simulink library "inp"  (R2021b)
settings: Solver=VariableStepAuto  StartTime=0.0  StopTime=10.0  RelTol=1e-3
undefined symbols (not defined in the file): C_TASK_5MS_S, FALSE, KINP_AcoreReadyToSlp_flg_ovrdflg, KINP_AcoreReadyToSlp_flg_ovrdval, KINP_AllowMovThd_OTA_enum_ovrdflg, KINP_AllowMovThd_OTA_enum_ovrdval, KINP_APSAngleTarget_Deg_ovrdflg, KINP_APSAngleTarget_Deg_ovrdval, KINP_APSDecReq_mps2_ovrdflg, KINP_APSDecReq_mps2_ovrdval, KINP_APSDecReqA_flg_ovrdflg, KINP_APSDecReqA_flg_ovrdval, KINP_APSDFLL_cm_ovrdflg, KINP_APSDFLL_cm_ovrdval, KINP_APSDFLR_cm_ovrdflg, KINP_APSDFLR_cm_ovrdval, KINP_APSDRLL_cm_ovrdflg, KINP_APSDRLL_cm_ovrdval, KINP_APSDRLR_cm_ovrdflg, KINP_APSDRLR_cm_ovrdval, KINP_APSExitCondition_enum_ovrdflg, KINP_APSExitCondition_enum_ovrdval, KINP_APSHWVer_enum_ovrdflg, KINP_APSHWVer_enum_ovrdval, KINP_APSProgressPCT_pct_ovrdflg, KINP_APSProgressPCT_pct_ovrdval, KINP_APSReq_enum_ovrdflg, KINP_APSReq_enum_ovrdval, KINP_APSRQDisplay_enum_ovrdflg, KINP_APSRQDisplay_enum_ovrdval, KINP_APSRqEPASCtrl_flg_ovrdflg, KINP_APSRqEPASCtrl_flg_ovrdval, KINP_APSShiftPosnReq_enum_ovrdval, KINP_APSShiftPosnReq_enum_ovrflg, KINP_APSSpeedCMD_kph_ovrdval, KINP_APSSpeedCMD_kph_ovrflg, KINP_APSStaSystem_enum_ovrdflg, KINP_APSStaSystem_enum_ovrdval, KINP_APSSWVer_enum_ovrdflg, KINP_APSSWVer_enum_ovrdval, KINP_APSVMCReqA_flg_ovrdval, KINP_APSVMCReqA_flg_ovrflg, KINP_APSVRqEPASCtrl_flg_ovrdflg, KINP_APSVRqEPASCtrl_flg_ovrdval, KINP_AuxBattVolmV_mV_ovrdflg, KINP_AuxBattVolmV_mV_ovrdval, KINP_CAASSta_enum_ovrdflg, KINP_CAASSta_enum_ovrdval, KINP_CAASVMCReqA_flg_ovrdval, KINP_CAASVMCReqA_flg_ovrflg, KINP_Chime_enum_ovrdflg, KINP_Chime_enum_ovrdval, KINP_ClearDTCcmd_flg_ovrdflg, KINP_ClearDTCcmd_flg_ovrdval, KINP_EvccAplusPwrUpReq_flg_ovrdflg, KINP_EvccAplusPwrUpReq_flg_ovrdval, KINP_LFID_raw_ovrdval, KINP_LFID_raw_ovrflg, KINP_LRID_raw_ovrdval, KINP_MemOffsetAccX_raw16_ovrdflg ... (+118)
libraries: FVT_lib x595, hcu_lib x1
(part 22 of 27)

== system inp/INP/CAN3/SignalCheck/MCU_R2 ==
  BHAL_outputs : Inport
  inp_CanValid_bus : Inport  Port=2
  RrCoolanttempReq : FVT_lib/inp/can_signal_template  SystemSampleTime=-1  VariantActivationTime=update diagram  Latency=0  AutoFrameSizeCalculation=off
      link override defval: Value=KINP_RrCoolanttempReq_cnt_defval
      link override fftdec: Value=KINP_RrCoolanttempReq_cnt_fftdec
      link override fftinc: Value=KINP_RrCoolanttempReq_cnt_fftinc
      link override fftlim: Value=KINP_RrCoolanttempReq_cnt_fftlim
      link override invalid: Value=KINP_RrCoolanttempReq_cnt_invalid
      link override ovrdflg: Value=KINP_RrCoolanttempReq_cnt_ovrdflg
      link override ovrdval: Value=KINP_RrCoolanttempReq_cnt_ovrdval
      link override setvalid: Value=KINP_RrCoolanttempReq_cnt_setvalid
      link override srvcflg: Value=KINP_RrCoolanttempReq_cnt_srvcflg
      link override srvcval: Value=KINP_RrCoolanttempReq_cnt_srvcval
  RrEOPSpdSet : FVT_lib/inp/can_signal_template  SystemSampleTime=-1  VariantActivationTime=update diagram  Latency=0  AutoFrameSizeCalculation=off
      link override defval: Value=KINP_RrEOPSpdSet_rpm_defval
      link override fftdec: Value=KINP_RrEOPSpdSet_rpm_fftdec
      link override fftinc: Value=KINP_RrEOPSpdSet_rpm_fftinc
      link override fftlim: Value=KINP_RrEOPSpdSet_rpm_fftlim
      link override invalid: Value=KINP_RrEOPSpdSet_rpm_invalid
      link override ovrdflg: Value=KINP_RrEOPSpdSet_rpm_ovrdflg
      link override ovrdval: Value=KINP_RrEOPSpdSet_rpm_ovrdval
      link override setvalid: Value=KINP_RrEOPSpdSet_rpm_setvalid
      link override srvcflg: Value=KINP_RrEOPSpdSet_rpm_srvcflg
      link override srvcval: Value=KINP_RrEOPSpdSet_rpm_srvcval
  RrFailcode1 : FVT_lib/inp/can_signal_template  SystemSampleTime=-1  VariantActivationTime=update diagram  Latency=0  AutoFrameSizeCalculation=off
      link override defval: Value=KINP_RrFailcode1_enum_defval
      link override fftdec: Value=KINP_RrFailcode1_enum_fftdec
      link override fftinc: Value=KINP_RrFailcode1_enum_fftinc
      link override fftlim: Value=KINP_RrFailcode1_enum_fftlim
      link override invalid: Value=KINP_RrFailcode1_enum_invalid
      link override ovrdflg: Value=KINP_RrFailcode1_enum_ovrdflg
      link override ovrdval: Value=KINP_RrFailcode1_enum_ovrdval
      link override setvalid: Value=KINP_RrFailcode1_enum_setvalid
      link override srvcflg: Value=KINP_RrFailcode1_enum_srvcflg
      link override srvcval: Value=KINP_RrFailcode1_enum_srvcval
  RrFailcode2 : FVT_lib/inp/can_signal_template  SystemSampleTime=-1  VariantActivationTime=update diagram  Latency=0  AutoFrameSizeCalculation=off
      link override defval: Value=KINP_RrFailcode2_enum_defval
      link override fftdec: Value=KINP_RrFailcode2_enum_fftdec
      link override fftinc: Value=KINP_RrFailcode2_enum_fftinc
      link override fftlim: Value=KINP_RrFailcode2_enum_fftlim
      link override invalid: Value=KINP_RrFailcode2_enum_invalid
      link override ovrdflg: Value=KINP_RrFailcode2_enum_ovrdflg
      link override ovrdval: Value=KINP_RrFailcode2_enum_ovrdval
      link override setvalid: Value=KINP_RrFailcode2_enum_setvalid
      link override srvcflg: Value=KINP_RrFailcode2_enum_srvcflg
      link override srvcval: Value=KINP_RrFailcode2_enum_srvcval
  RrFailcodehistory1 : FVT_lib/inp/can_signal_template  SystemSampleTime=-1  VariantActivationTime=update diagram  Latency=0  AutoFrameSizeCalculation=off
      link override defval: Value=KINP_RrFailcodehistory1_enum_defval
      link override fftdec: Value=KINP_RrFailcodehistory1_enum_fftdec
      link override fftinc: Value=KINP_RrFailcodehistory1_enum_fftinc
      link override fftlim: Value=KINP_RrFailcodehistory1_enum_fftlim
      link override invalid: Value=KINP_RrFailcodehistory1_enum_invalid
      link override ovrdflg: Value=KINP_RrFailcodehistory1_enum_ovrdflg
      link override ovrdval: Value=KINP_RrFailcodehistory1_enum_ovrdval
      link override setvalid: Value=KINP_RrFailcodehistory1_enum_setvalid
      link override srvcflg: Value=KINP_RrFailcodehistory1_enum_srvcflg
      link override srvcval: Value=KINP_RrFailcodehistory1_enum_srvcval
  RrFailcodehistory2 : FVT_lib/inp/can_signal_template  SystemSampleTime=-1  VariantActivationTime=update diagram  Latency=0  AutoFrameSizeCalculation=off
      link override defval: Value=KINP_RrFailcodehistory2_enum_defval
      link override fftdec: Value=KINP_RrFailcodehistory2_enum_fftdec
      link override fftinc: Value=KINP_RrFailcodehistory2_enum_fftinc
      link override fftlim: Value=KINP_RrFailcodehistory2_enum_fftlim
      link override invalid: Value=KINP_RrFailcodehistory2_enum_invalid
      link override ovrdflg: Value=KINP_RrFailcodehistory2_enum_ovrdflg
      link override ovrdval: Value=KINP_RrFailcodehistory2_enum_ovrdval
      link override setvalid: Value=KINP_RrFailcodehistory2_enum_setvalid
      link override srvcflg: Value=KINP_RrFailcodehistory2_enum_srvcflg
      link override srvcval: Value=KINP_RrFailcodehistory2_enum_srvcval
  RrLLCTemp : FVT_lib/inp/can_signal_template  SystemSampleTime=-1  VariantActivationTime=update diagram  Latency=0  AutoFrameSizeCalculation=off
      link override defval: Value=KINP_RrLLCTemp_C_defval
      link override fftdec: Value=KINP_RrLLCTemp_C_fftdec
      link override fftinc: Value=KINP_RrLLCTemp_C_fftinc
      link override fftlim: Value=KINP_RrLLCTemp_C_fftlim
      link override invalid: Value=KINP_RrLLCTemp_C_invalid
      link override ovrdflg: Value=KINP_RrLLCTemp_C_ovrdflg
      link override ovrdval: Value=KINP_RrLLCTemp_C_ovrdval
      link override setvalid: Value=KINP_RrLLCTemp_C_setvalid
      link override srvcflg: Value=KINP_RrLLCTemp_C_srvcflg
      link override srvcval: Value=KINP_RrLLCTemp_C_srvcval
  RrLLCflowReq : FVT_lib/inp/can_signal_template  SystemSampleTime=-1  VariantActivationTime=update diagram  Latency=0  AutoFrameSizeCalculation=off
      link override defval: Value=KINP_RrLLCflowReq_Lpmin_defval
      link override fftdec: Value=KINP_RrLLCflowReq_Lpmin_fftdec
      link override fftinc: Value=KINP_RrLLCflowReq_Lpmin_fftinc
      link override fftlim: Value=KINP_RrLLCflowReq_Lpmin_fftlim
      link override invalid: Value=KINP_RrLLCflowReq_Lpmin_invalid
      link override ovrdflg: Value=KINP_RrLLCflowReq_Lpmin_ovrdflg
      link override ovrdval: Value=KINP_RrLLCflowReq_Lpmin_ovrdval
      link override setvalid: Value=KINP_RrLLCflowReq_Lpmin_setvalid
      link override srvcflg: Value=KINP_RrLLCflowReq_Lpmin_srvcflg
      link override srvcval: Value=KINP_RrLLCflowReq_Lpmin_srvcval
  RrMCUTempWarn : FVT_lib/inp/can_signal_template  SystemSampleTime=-1  VariantActivationTime=update diagram  Latency=0  AutoFrameSizeCalculation=off
      link override defval: Value=KINP_RrMCUTempWarn_enum_defval
      link override fftdec: Value=KINP_RrMCUTempWarn_enum_fftdec
      link override fftinc: Value=KINP_RrMCUTempWarn_enum_fftinc
      link override fftlim: Value=KINP_RrMCUTempWarn_enum_fftlim
      link override invalid: Value=KINP_RrMCUTempWarn_enum_invalid
      link override ovrdflg: Value=KINP_RrMCUTempWarn_enum_ovrdflg
      link override ovrdval: Value=KINP_RrMCUTempWarn_enum_ovrdval
      link override setvalid: Value=KINP_RrMCUTempWarn_enum_setvalid
      link override srvcflg: Value=KINP_RrMCUTempWarn_enum_srvcflg
      link override srvcval: Value=KINP_RrMCUTempWarn_enum_srvcval
  RrTMTempWarn : FVT_lib/inp/can_signal_template  SystemSampleTime=-1  VariantActivationTime=update diagram  Latency=0  AutoFrameSizeCalculation=off
      link override defval: Value=KINP_RrTMTempWarn_enum_defval
      link override fftdec: Value=KINP_RrTMTempWarn_enum_fftdec
      link override fftinc: Value=KINP_RrTMTempWarn_enum_fftinc
      link override fftlim: Value=KINP_RrTMTempWarn_enum_fftlim
      link override invalid: Value=KINP_RrTMTempWarn_enum_invalid
      link override ovrdflg: Value=KINP_RrTMTempWarn_enum_ovrdflg
      link override ovrdval: Value=KINP_RrTMTempWarn_enum_ovrdval
      link override setvalid: Value=KINP_RrTMTempWarn_enum_setvalid
      link override srvcflg: Value=KINP_RrTMTempWarn_enum_srvcflg
      link override srvcval: Value=KINP_RrTMTempWarn_enum_srvcval
  Terminator_{1..10} (10 alike) : Terminator
  True_VHAL_RrCoolanttempReq_cnt : Constant  Value=TRUE  OutDataTypeStr=boolean
  True_VHAL_RrEOPSpdSet_rpm : Constant  Value=TRUE  OutDataTypeStr=boolean
  True_VHAL_RrFailcode1_enum : Constant  Value=TRUE  OutDataTypeStr=boolean
  True_VHAL_RrFailcode2_enum : Constant  Value=TRUE  OutDataTypeStr=boolean
  True_VHAL_RrFailcodehistory1_enum : Constant  Value=TRUE  OutDataTypeStr=boolean
  True_VHAL_RrFailcodehistory2_enum : Constant  Value=TRUE  OutDataTypeStr=boolean
  True_VHAL_RrLLCTemp_C : Constant  Value=TRUE  OutDataTypeStr=boolean
  True_VHAL_RrLLCflowReq_Lpmin : Constant  Value=TRUE  OutDataTypeStr=boolean
  True_VHAL_RrMCUTempWarn_enum : Constant  Value=TRUE  OutDataTypeStr=boolean
  True_VHAL_RrTMTempWarn_enum : Constant  Value=TRUE  OutDataTypeStr=boolean
  slr1_{1..10} (10 alike) : BusSelector  OutputSignals=VINP_CANMsgValidMCUR2_flg
  slr_VHAL_RrCoolanttempReq_cnt : BusSelector  OutputSignals=VHAL_RrCoolanttempReq_cnt
  slr_VHAL_RrEOPSpdSet_rpm : BusSelector  OutputSignals=VHAL_RrEOPSpdSet_rpm
  slr_VHAL_RrFailcode1_enum : BusSelector  OutputSignals=VHAL_RrFailcode1_enum
  slr_VHAL_RrFailcode2_enum : BusSelector  OutputSignals=VHAL_RrFailcode2_enum
  slr_VHAL_RrFailcodehistory1_enum : BusSelector  OutputSignals=VHAL_RrFailcodehistory1_enum
  slr_VHAL_RrFailcodehistory2_enum : BusSelector  OutputSignals=VHAL_RrFailcodehistory2_enum
  slr_VHAL_RrLLCTemp_C : BusSelector  OutputSignals=VHAL_RrLLCTemp_C
  slr_VHAL_RrLLCflowReq_Lpmin : BusSelector  OutputSignals=VHAL_RrLLCflowReq_Lpmin
  slr_VHAL_RrMCUTempWarn_enum : BusSelector  OutputSignals=VHAL_RrMCUTempWarn_enum
  slr_VHAL_RrTMTempWarn_enum : BusSelector  OutputSignals=VHAL_RrTMTempWarn_enum
  VINP_RrCoolanttempReq_cnt : Outport
  VINP_RrEOPSpdSet_rpm : Outport  Port=2
  VINP_RrFailcode1_enum : Outport  Port=3
  VINP_RrFailcode2_enum : Outport  Port=4
  VINP_RrFailcodehistory1_enum : Outport  Port=5
  VINP_RrFailcodehistory2_enum : Outport  Port=6
  VINP_RrLLCTemp_C : Outport  Port=7
  VINP_RrLLCflowReq_Lpmin : Outport  Port=8
  VINP_RrMCUTempWarn_enum : Outport  Port=9
  VINP_RrTMTempWarn_enum : Outport  Port=10
  wires:
  BHAL_outputs/1 -> [BHAL_outputs]
  inp_CanValid_bus/1 -> [inp_CanValid_bus]
  [BHAL_outputs] -> slr_VHAL_RrCoolanttempReq_cnt/1
  slr_VHAL_RrCoolanttempReq_cnt/1 -> RrCoolanttempReq/1  "<VHAL_RrCoolanttempReq_cnt>"
  True_VHAL_RrCoolanttempReq_cnt/1 -> RrCoolanttempReq/2
  [inp_CanValid_bus] -> slr1_1/1
  slr1_1/1 -> RrCoolanttempReq/3  "<VINP_CANMsgValidMCUR2_flg>"
  RrCoolanttempReq/1 -> VINP_RrCoolanttempReq_cnt/1  "VINP_RrCoolanttempReq_cnt"
  RrCoolanttempReq/2 -> Terminator_1/1
  [BHAL_outputs] -> slr_VHAL_RrEOPSpdSet_rpm/1
  slr_VHAL_RrEOPSpdSet_rpm/1 -> RrEOPSpdSet/1  "<VHAL_RrEOPSpdSet_rpm>"
  True_VHAL_RrEOPSpdSet_rpm/1 -> RrEOPSpdSet/2
  [inp_CanValid_bus] -> slr1_2/1
  slr1_2/1 -> RrEOPSpdSet/3  "<VINP_CANMsgValidMCUR2_flg>"
  RrEOPSpdSet/1 -> VINP_RrEOPSpdSet_rpm/1  "VINP_RrEOPSpdSet_rpm"
  RrEOPSpdSet/2 -> Terminator_2/1
  [BHAL_outputs] -> slr_VHAL_RrFailcode1_enum/1
  slr_VHAL_RrFailcode1_enum/1 -> RrFailcode1/1  "<VHAL_RrFailcode1_enum>"
  True_VHAL_RrFailcode1_enum/1 -> RrFailcode1/2
  [inp_CanValid_bus] -> slr1_3/1
  slr1_3/1 -> RrFailcode1/3  "<VINP_CANMsgValidMCUR2_flg>"
  RrFailcode1/1 -> VINP_RrFailcode1_enum/1  "VINP_RrFailcode1_enum"
  RrFailcode1/2 -> Terminator_3/1
  [BHAL_outputs] -> slr_VHAL_RrFailcode2_enum/1
  slr_VHAL_RrFailcode2_enum/1 -> RrFailcode2/1  "<VHAL_RrFailcode2_enum>"
  True_VHAL_RrFailcode2_enum/1 -> RrFailcode2/2
  [inp_CanValid_bus] -> slr1_4/1
  slr1_4/1 -> RrFailcode2/3  "<VINP_CANMsgValidMCUR2_flg>"
  RrFailcode2/1 -> VINP_RrFailcode2_enum/1  "VINP_RrFailcode2_enum"
  RrFailcode2/2 -> Terminator_4/1
  [BHAL_outputs] -> slr_VHAL_RrFailcodehistory1_enum/1
  slr_VHAL_RrFailcodehistory1_enum/1 -> RrFailcodehistory1/1  "<VHAL_RrFailcodehistory1_enum>"
  True_VHAL_RrFailcodehistory1_enum/1 -> RrFailcodehistory1/2
  [inp_CanValid_bus] -> slr1_5/1
  slr1_5/1 -> RrFailcodehistory1/3  "<VINP_CANMsgValidMCUR2_flg>"
  RrFailcodehistory1/1 -> VINP_RrFailcodehistory1_enum/1  "VINP_RrFailcodehistory1_enum"
  RrFailcodehistory1/2 -> Terminator_5/1
  [BHAL_outputs] -> slr_VHAL_RrFailcodehistory2_enum/1
  slr_VHAL_RrFailcodehistory2_enum/1 -> RrFailcodehistory2/1  "<VHAL_RrFailcodehistory2_enum>"
  True_VHAL_RrFailcodehistory2_enum/1 -> RrFailcodehistory2/2
  [inp_CanValid_bus] -> slr1_6/1
  slr1_6/1 -> RrFailcodehistory2/3  "<VINP_CANMsgValidMCUR2_flg>"
  RrFailcodehistory2/1 -> VINP_RrFailcodehistory2_enum/1  "VINP_RrFailcodehistory2_enum"
  RrFailcodehistory2/2 -> Terminator_6/1
  [BHAL_outputs] -> slr_VHAL_RrLLCTemp_C/1
  slr_VHAL_RrLLCTemp_C/1 -> RrLLCTemp/1  "<VHAL_RrLLCTemp_C>"
  True_VHAL_RrLLCTemp_C/1 -> RrLLCTemp/2
  [inp_CanValid_bus] -> slr1_7/1
  slr1_7/1 -> RrLLCTemp/3  "<VINP_CANMsgValidMCUR2_flg>"
  RrLLCTemp/1 -> VINP_RrLLCTemp_C/1  "VINP_RrLLCTemp_C"
  RrLLCTemp/2 -> Terminator_7/1
  [BHAL_outputs] -> slr_VHAL_RrLLCflowReq_Lpmin/1
  slr_VHAL_RrLLCflowReq_Lpmin/1 -> RrLLCflowReq/1  "<VHAL_RrLLCflowReq_Lpmin>"
  True_VHAL_RrLLCflowReq_Lpmin/1 -> RrLLCflowReq/2
  [inp_CanValid_bus] -> slr1_8/1
  slr1_8/1 -> RrLLCflowReq/3  "<VINP_CANMsgValidMCUR2_flg>"
  RrLLCflowReq/1 -> VINP_RrLLCflowReq_Lpmin/1  "VINP_RrLLCflowReq_Lpmin"
  RrLLCflowReq/2 -> Terminator_8/1
  [BHAL_outputs] -> slr_VHAL_RrMCUTempWarn_enum/1
  slr_VHAL_RrMCUTempWarn_enum/1 -> RrMCUTempWarn/1  "<VHAL_RrMCUTempWarn_enum>"
  True_VHAL_RrMCUTempWarn_enum/1 -> RrMCUTempWarn/2
  [inp_CanValid_bus] -> slr1_9/1
  slr1_9/1 -> RrMCUTempWarn/3  "<VINP_CANMsgValidMCUR2_flg>"
  RrMCUTempWarn/1 -> VINP_RrMCUTempWarn_enum/1  "VINP_RrMCUTempWarn_enum"
  RrMCUTempWarn/2 -> Terminator_9/1
  [BHAL_outputs] -> slr_VHAL_RrTMTempWarn_enum/1
  slr_VHAL_RrTMTempWarn_enum/1 -> RrTMTempWarn/1  "<VHAL_RrTMTempWarn_enum>"
  True_VHAL_RrTMTempWarn_enum/1 -> RrTMTempWarn/2
  [inp_CanValid_bus] -> slr1_10/1
  slr1_10/1 -> RrTMTempWarn/3  "<VINP_CANMsgValidMCUR2_flg>"
  RrTMTempWarn/1 -> VINP_RrTMTempWarn_enum/1  "VINP_RrTMTempWarn_enum"
  RrTMTempWarn/2 -> Terminator_10/1

== system inp/INP/CAN3/SignalCheck/Shifter1 ==
  BHAL_outputs : Inport
  inp_CanValid_bus : Inport  Port=2
  Shifter1CSErr : FVT_lib/inp/can_signal_template  SystemSampleTime=-1  VariantActivationTime=update diagram  Latency=0  AutoFrameSizeCalculation=off
      link override defval: Value=KINP_Shifter1CSErr_flg_defval
      link override fftdec: Value=KINP_Shifter1CSErr_flg_fftdec
      link override fftinc: Value=KINP_Shifter1CSErr_flg_fftinc
      link override fftlim: Value=KINP_Shifter1CSErr_flg_fftlim
      link override invalid: Value=KINP_Shifter1CSErr_flg_invalid
      link override ovrdflg: Value=KINP_Shifter1CSErr_flg_ovrdflg
      link override ovrdval: Value=KINP_Shifter1CSErr_flg_ovrdval
      link override setvalid: Value=KINP_Shifter1CSErr_flg_setvalid
      link override srvcflg: Value=KINP_Shifter1CSErr_flg_srvcflg
      link override srvcval: Value=KINP_Shifter1CSErr_flg_srvcval
  Shifter1RCErr : FVT_lib/inp/can_signal_template  SystemSampleTime=-1  VariantActivationTime=update diagram  Latency=0  AutoFrameSizeCalculation=off
      link override defval: Value=KINP_Shifter1RCErr_flg_defval
      link override fftdec: Value=KINP_Shifter1RCErr_flg_fftdec
      link override fftinc: Value=KINP_Shifter1RCErr_flg_fftinc
      link override fftlim: Value=KINP_Shifter1RCErr_flg_fftlim
      link override invalid: Value=KINP_Shifter1RCErr_flg_invalid
      link override ovrdflg: Value=KINP_Shifter1RCErr_flg_ovrdflg
      link override ovrdval: Value=KINP_Shifter1RCErr_flg_ovrdval
      link override setvalid: Value=KINP_Shifter1RCErr_flg_setvalid
      link override srvcflg: Value=KINP_Shifter1RCErr_flg_srvcflg
      link override srvcval: Value=KINP_Shifter1RCErr_flg_srvcval
  ShifterCRC8 : FVT_lib/inp/can_signal_template  SystemSampleTime=-1  VariantActivationTime=update diagram  Latency=0  AutoFrameSizeCalculation=off
      link override defval: Value=KINP_ShifterCRC8_enum_defval
      link override fftdec: Value=KINP_ShifterCRC8_enum_fftdec
      link override fftinc: Value=KINP_ShifterCRC8_enum_fftinc
      link override fftlim: Value=KINP_ShifterCRC8_enum_fftlim
      link override invalid: Value=KINP_ShifterCRC8_enum_invalid
      link override ovrdflg: Value=KINP_ShifterCRC8_enum_ovrdflg
      link override ovrdval: Value=KINP_ShifterCRC8_enum_ovrdval
      link override setvalid: Value=KINP_ShifterCRC8_enum_setvalid
      link override srvcflg: Value=KINP_ShifterCRC8_enum_srvcflg
      link override srvcval: Value=KINP_ShifterCRC8_enum_srvcval
  ShifterHandleCmd : FVT_lib/inp/can_signal_template  SystemSampleTime=-1  VariantActivationTime=update diagram  Latency=0  AutoFrameSizeCalculation=off
      link override defval: Value=KINP_ShifterHandleCmd_enum_defval
      link override fftdec: Value=KINP_ShifterHandleCmd_enum_fftdec
      link override fftinc: Value=KINP_ShifterHandleCmd_enum_fftinc
      link override fftlim: Value=KINP_ShifterHandleCmd_enum_fftlim
      link override invalid: Value=KINP_ShifterHandleCmd_enum_invalid
      link override ovrdflg: Value=KINP_ShifterHandleCmd_enum_ovrdflg
      link override ovrdval: Value=KINP_ShifterHandleCmd_enum_ovrdval
      link override setvalid: Value=KINP_ShifterHandleCmd_enum_setvalid
      link override srvcflg: Value=KINP_ShifterHandleCmd_enum_srvcflg
      link override srvcval: Value=KINP_ShifterHandleCmd_enum_srvcval
  ShifterRC : FVT_lib/inp/can_signal_template  SystemSampleTime=-1  VariantActivationTime=update diagram  Latency=0  AutoFrameSizeCalculation=off
      link override defval: Value=KINP_ShifterRC_enum_defval
      link override fftdec: Value=KINP_ShifterRC_enum_fftdec
      link override fftinc: Value=KINP_ShifterRC_enum_fftinc
      link override fftlim: Value=KINP_ShifterRC_enum_fftlim
      link override invalid: Value=KINP_ShifterRC_enum_invalid
      link override ovrdflg: Value=KINP_ShifterRC_enum_ovrdflg
      link override ovrdval: Value=KINP_ShifterRC_enum_ovrdval
      link override setvalid: Value=KINP_ShifterRC_enum_setvalid
      link override srvcflg: Value=KINP_ShifterRC_enum_srvcflg
      link override srvcval: Value=KINP_ShifterRC_enum_srvcval
  Terminator_{1..5} (5 alike) : Terminator
  True_VHAL_Shifter1CSErr_flg : Constant  Value=TRUE  OutDataTypeStr=boolean
  True_VHAL_Shifter1RCErr_flg : Constant  Value=TRUE  OutDataTypeStr=boolean
  True_VHAL_ShifterCRC8_enum : Constant  Value=TRUE  OutDataTypeStr=boolean
  True_VHAL_ShifterHandleCmd_enum : Constant  Value=TRUE  OutDataTypeStr=boolean
  True_VHAL_ShifterRC_enum : Constant  Value=TRUE  OutDataTypeStr=boolean
  slr1_{1..5} (5 alike) : BusSelector  OutputSignals=VINP_CANMsgValidShifter1_flg
  slr_VHAL_Shifter1CSErr_flg : BusSelector  OutputSignals=VHAL_Shifter1CSErr_flg
  slr_VHAL_Shifter1RCErr_flg : BusSelector  OutputSignals=VHAL_Shifter1RCErr_flg
  slr_VHAL_ShifterCRC8_enum : BusSelector  OutputSignals=VHAL_ShifterCRC8_enum
  slr_VHAL_ShifterHandleCmd_enum : BusSelector  OutputSignals=VHAL_ShifterHandleCmd_enum
  slr_VHAL_ShifterRC_enum : BusSelector  OutputSignals=VHAL_ShifterRC_enum
  VINP_Shifter1CSErr_flg : Outport
  VINP_Shifter1RCErr_flg : Outport  Port=2
  VINP_ShifterCRC8_enum : Outport  Port=3
  VINP_ShifterHandleCmd_enum : Outport  Port=4
  VINP_ShifterRC_enum : Outport  Port=5
  wires:
  BHAL_outputs/1 -> [BHAL_outputs]
  inp_CanValid_bus/1 -> [inp_CanValid_bus]
  [BHAL_outputs] -> slr_VHAL_Shifter1CSErr_flg/1
  slr_VHAL_Shifter1CSErr_flg/1 -> Shifter1CSErr/1  "<VHAL_Shifter1CSErr_flg>"
  True_VHAL_Shifter1CSErr_flg/1 -> Shifter1CSErr/2
  [inp_CanValid_bus] -> slr1_1/1
  slr1_1/1 -> Shifter1CSErr/3  "<VINP_CANMsgValidShifter1_flg>"
  Shifter1CSErr/1 -> VINP_Shifter1CSErr_flg/1  "VINP_Shifter1CSErr_flg"
  Shifter1CSErr/2 -> Terminator_1/1
  [BHAL_outputs] -> slr_VHAL_Shifter1RCErr_flg/1
  slr_VHAL_Shifter1RCErr_flg/1 -> Shifter1RCErr/1  "<VHAL_Shifter1RCErr_flg>"
  True_VHAL_Shifter1RCErr_flg/1 -> Shifter1RCErr/2
  [inp_CanValid_bus] -> slr1_2/1
  slr1_2/1 -> Shifter1RCErr/3  "<VINP_CANMsgValidShifter1_flg>"
  Shifter1RCErr/1 -> VINP_Shifter1RCErr_flg/1  "VINP_Shifter1RCErr_flg"
  Shifter1RCErr/2 -> Terminator_2/1
  [BHAL_outputs] -> slr_VHAL_ShifterCRC8_enum/1
  slr_VHAL_ShifterCRC8_enum/1 -> ShifterCRC8/1  "<VHAL_ShifterCRC8_enum>"
  True_VHAL_ShifterCRC8_enum/1 -> ShifterCRC8/2
  [inp_CanValid_bus] -> slr1_3/1
  slr1_3/1 -> ShifterCRC8/3  "<VINP_CANMsgValidShifter1_flg>"
  ShifterCRC8/1 -> VINP_ShifterCRC8_enum/1  "VINP_ShifterCRC8_enum"
  ShifterCRC8/2 -> Terminator_3/1
  [BHAL_outputs] -> slr_VHAL_ShifterHandleCmd_enum/1
  slr_VHAL_ShifterHandleCmd_enum/1 -> ShifterHandleCmd/1  "<VHAL_ShifterHandleCmd_enum>"
  True_VHAL_ShifterHandleCmd_enum/1 -> ShifterHandleCmd/2
  [inp_CanValid_bus] -> slr1_4/1
  slr1_4/1 -> ShifterHandleCmd/3  "<VINP_CANMsgValidShifter1_flg>"
  ShifterHandleCmd/1 -> VINP_ShifterHandleCmd_enum/1  "VINP_ShifterHandleCmd_enum"
  ShifterHandleCmd/2 -> Terminator_4/1
  [BHAL_outputs] -> slr_VHAL_ShifterRC_enum/1
  slr_VHAL_ShifterRC_enum/1 -> ShifterRC/1  "<VHAL_ShifterRC_enum>"
  True_VHAL_ShifterRC_enum/1 -> ShifterRC/2
  [inp_CanValid_bus] -> slr1_5/1
  slr1_5/1 -> ShifterRC/3  "<VINP_CANMsgValidShifter1_flg>"
  ShifterRC/1 -> VINP_ShifterRC_enum/1  "VINP_ShifterRC_enum"
  ShifterRC/2 -> Terminator_5/1

== system inp/INP/CAN4/SignalCheck/DKC1 ==
  BHAL_outputs : Inport
  inp_CanValid_bus : Inport  Port=2
  DKCReVehData : FVT_lib/inp/can_signal_template  SystemSampleTime=-1  VariantActivationTime=update diagram  Latency=0  AutoFrameSizeCalculation=off
      link override defval: Value=KINP_DKCReVehData_enum_defval
      link override fftdec: Value=KINP_DKCReVehData_enum_fftdec
      link override fftinc: Value=KINP_DKCReVehData_enum_fftinc
      link override fftlim: Value=KINP_DKCReVehData_enum_fftlim
      link override invalid: Value=KINP_DKCReVehData_enum_invalid
      link override ovrdflg: Value=KINP_DKCReVehData_enum_ovrdflg
      link override ovrdval: Value=KINP_DKCReVehData_enum_ovrdval
      link override setvalid: Value=KINP_DKCReVehData_enum_setvalid
      link override srvcflg: Value=KINP_DKCReVehData_enum_srvcflg
      link override srvcval: Value=KINP_DKCReVehData_enum_srvcval
  DKCRemotePW : FVT_lib/inp/can_signal_template  SystemSampleTime=-1  VariantActivationTime=update diagram  Latency=0  AutoFrameSizeCalculation=off
      link override defval: Value=KINP_DKCRemotePW_enum_defval
      link override fftdec: Value=KINP_DKCRemotePW_enum_fftdec
      link override fftinc: Value=KINP_DKCRemotePW_enum_fftinc
      link override fftlim: Value=KINP_DKCRemotePW_enum_fftlim
      link override invalid: Value=KINP_DKCRemotePW_enum_invalid
      link override ovrdflg: Value=KINP_DKCRemotePW_enum_ovrdflg
      link override ovrdval: Value=KINP_DKCRemotePW_enum_ovrdval
      link override setvalid: Value=KINP_DKCRemotePW_enum_setvalid
      link override srvcflg: Value=KINP_DKCRemotePW_enum_srvcflg
      link override srvcval: Value=KINP_DKCRemotePW_enum_srvcval
  PCommandToBCM : FVT_lib/inp/can_signal_template  SystemSampleTime=-1  VariantActivationTime=update diagram  Latency=0  AutoFrameSizeCalculation=off
      link override defval: Value=KINP_PCommandToBCM_enum_defval
      link override fftdec: Value=KINP_PCommandToBCM_enum_fftdec
      link override fftinc: Value=KINP_PCommandToBCM_enum_fftinc
      link override fftlim: Value=KINP_PCommandToBCM_enum_fftlim
      link override invalid: Value=KINP_PCommandToBCM_enum_invalid
      link override ovrdflg: Value=KINP_PCommandToBCM_enum_ovrdflg
      link override ovrdval: Value=KINP_PCommandToBCM_enum_ovrdval
      link override setvalid: Value=KINP_PCommandToBCM_enum_setvalid
      link override srvcflg: Value=KINP_PCommandToBCM_enum_srvcflg
      link override srvcval: Value=KINP_PCommandToBCM_enum_srvcval
  PCommandToPTG : FVT_lib/inp/can_signal_template  SystemSampleTime=-1  VariantActivationTime=update diagram  Latency=0  AutoFrameSizeCalculation=off
      link override defval: Value=KINP_PCommandToPTG_enum_defval
      link override fftdec: Value=KINP_PCommandToPTG_enum_fftdec
      link override fftinc: Value=KINP_PCommandToPTG_enum_fftinc
      link override fftlim: Value=KINP_PCommandToPTG_enum_fftlim
      link override invalid: Value=KINP_PCommandToPTG_enum_invalid
      link override ovrdflg: Value=KINP_PCommandToPTG_enum_ovrdflg
      link override ovrdval: Value=KINP_PCommandToPTG_enum_ovrdval
      link override setvalid: Value=KINP_PCommandToPTG_enum_setvalid
      link override srvcflg: Value=KINP_PCommandToPTG_enum_srvcflg
      link override srvcval: Value=KINP_PCommandToPTG_enum_srvcval
  PDKeyAreaLockUnlock : FVT_lib/inp/can_signal_template  SystemSampleTime=-1  VariantActivationTime=update diagram  Latency=0  AutoFrameSizeCalculation=off
      link override defval: Value=KINP_PDKeyAreaLockUnlock_enum_defval
      link override fftdec: Value=KINP_PDKeyAreaLockUnlock_enum_fftdec
      link override fftinc: Value=KINP_PDKeyAreaLockUnlock_enum_fftinc
      link override fftlim: Value=KINP_PDKeyAreaLockUnlock_enum_fftlim
      link override invalid: Value=KINP_PDKeyAreaLockUnlock_enum_invalid
      link override ovrdflg: Value=KINP_PDKeyAreaLockUnlock_enum_ovrdflg
      link override ovrdval: Value=KINP_PDKeyAreaLockUnlock_enum_ovrdval
      link override setvalid: Value=KINP_PDKeyAreaLockUnlock_enum_setvalid
      link override srvcflg: Value=KINP_PDKeyAreaLockUnlock_enum_srvcflg
      link override srvcval: Value=KINP_PDKeyAreaLockUnlock_enum_srvcval
  PDKeyAreaPS : FVT_lib/inp/can_signal_template  SystemSampleTime=-1  VariantActivationTime=update diagram  Latency=0  AutoFrameSizeCalculation=off
      link override defval: Value=KINP_PDKeyAreaPS_enum_defval
      link override fftdec: Value=KINP_PDKeyAreaPS_enum_fftdec
      link override fftinc: Value=KINP_PDKeyAreaPS_enum_fftinc
      link override fftlim: Value=KINP_PDKeyAreaPS_enum_fftlim
      link override invalid: Value=KINP_PDKeyAreaPS_enum_invalid
      link override ovrdflg: Value=KINP_PDKeyAreaPS_enum_ovrdflg
      link override ovrdval: Value=KINP_PDKeyAreaPS_enum_ovrdval
      link override setvalid: Value=KINP_PDKeyAreaPS_enum_setvalid
      link override srvcflg: Value=KINP_PDKeyAreaPS_enum_srvcflg
      link override srvcval: Value=KINP_PDKeyAreaPS_enum_srvcval
  PDKeyAreaPTG : FVT_lib/inp/can_signal_template  SystemSampleTime=-1  VariantActivationTime=update diagram  Latency=0  AutoFrameSizeCalculation=off
      link override defval: Value=KINP_PDKeyAreaPTG_enum_defval
      link override fftdec: Value=KINP_PDKeyAreaPTG_enum_fftdec
      link override fftinc: Value=KINP_PDKeyAreaPTG_enum_fftinc
      link override fftlim: Value=KINP_PDKeyAreaPTG_enum_fftlim
      link override invalid: Value=KINP_PDKeyAreaPTG_enum_invalid
      link override ovrdflg: Value=KINP_PDKeyAreaPTG_enum_ovrdflg
      link override ovrdval: Value=KINP_PDKeyAreaPTG_enum_ovrdval
      link override setvalid: Value=KINP_PDKeyAreaPTG_enum_setvalid
      link override srvcflg: Value=KINP_PDKeyAreaPTG_enum_srvcflg
      link override srvcval: Value=KINP_PDKeyAreaPTG_enum_srvcval
  PDKeyWelcome : FVT_lib/inp/can_signal_template  SystemSampleTime=-1  VariantActivationTime=update diagram  Latency=0  AutoFrameSizeCalculation=off
      link override defval: Value=KINP_PDKeyWelcome_enum_defval
      link override fftdec: Value=KINP_PDKeyWelcome_enum_fftdec
      link override fftinc: Value=KINP_PDKeyWelcome_enum_fftinc
      link override fftlim: Value=KINP_PDKeyWelcome_enum_fftlim
      link override invalid: Value=KINP_PDKeyWelcome_enum_invalid
      link override ovrdflg: Value=KINP_PDKeyWelcome_enum_ovrdflg
      link override ovrdval: Value=KINP_PDKeyWelcome_enum_ovrdval
      link override setvalid: Value=KINP_PDKeyWelcome_enum_setvalid
      link override srvcflg: Value=KINP_PDKeyWelcome_enum_srvcflg
      link override srvcval: Value=KINP_PDKeyWelcome_enum_srvcval
  PDkeyShowIVI : FVT_lib/inp/can_signal_template  SystemSampleTime=-1  VariantActivationTime=update diagram  Latency=0  AutoFrameSizeCalculation=off
      link override defval: Value=KINP_PDkeyShowIVI_enum_defval
      link override fftdec: Value=KINP_PDkeyShowIVI_enum_fftdec
      link override fftinc: Value=KINP_PDkeyShowIVI_enum_fftinc
      link override fftlim: Value=KINP_PDkeyShowIVI_enum_fftlim
      link override invalid: Value=KINP_PDkeyShowIVI_enum_invalid
      link override ovrdflg: Value=KINP_PDkeyShowIVI_enum_ovrdflg
      link override ovrdval: Value=KINP_PDkeyShowIVI_enum_ovrdval
      link override setvalid: Value=KINP_PDkeyShowIVI_enum_setvalid
      link override srvcflg: Value=KINP_PDkeyShowIVI_enum_srvcflg
      link override srvcval: Value=KINP_PDkeyShowIVI_enum_srvcval
  PKeyMiss : FVT_lib/inp/can_signal_template  SystemSampleTime=-1  VariantActivationTime=update diagram  Latency=0  AutoFrameSizeCalculation=off
      link override defval: Value=KINP_PKeyMiss_flg_defval
      link override fftdec: Value=KINP_PKeyMiss_flg_fftdec
      link override fftinc: Value=KINP_PKeyMiss_flg_fftinc
      link override fftlim: Value=KINP_PKeyMiss_flg_fftlim
      link override invalid: Value=KINP_PKeyMiss_flg_invalid
      link override ovrdflg: Value=KINP_PKeyMiss_flg_ovrdflg
      link override ovrdval: Value=KINP_PKeyMiss_flg_ovrdval
      link override setvalid: Value=KINP_PKeyMiss_flg_setvalid
      link override srvcflg: Value=KINP_PKeyMiss_flg_srvcflg
      link override srvcval: Value=KINP_PKeyMiss_flg_srvcval
  PKeyMode : FVT_lib/inp/can_signal_template  SystemSampleTime=-1  VariantActivationTime=update diagram  Latency=0  AutoFrameSizeCalculation=off
      link override defval: Value=KINP_PKeyMode_enum_defval
      link override fftdec: Value=KINP_PKeyMode_enum_fftdec
      link override fftinc: Value=KINP_PKeyMode_enum_fftinc
      link override fftlim: Value=KINP_PKeyMode_enum_fftlim
      link override invalid: Value=KINP_PKeyMode_enum_invalid
      link override ovrdflg: Value=KINP_PKeyMode_enum_ovrdflg
      link override ovrdval: Value=KINP_PKeyMode_enum_ovrdval
      link override setvalid: Value=KINP_PKeyMode_enum_setvalid
      link override srvcflg: Value=KINP_PKeyMode_enum_srvcflg
      link override srvcval: Value=KINP_PKeyMode_enum_srvcval
  PUIDLowPower : FVT_lib/inp/can_signal_template  SystemSampleTime=-1  VariantActivationTime=update diagram  Latency=0  AutoFrameSizeCalculation=off
      link override defval: Value=KINP_PUIDLowPower_flg_defval
      link override fftdec: Value=KINP_PUIDLowPower_flg_fftdec
      link override fftinc: Value=KINP_PUIDLowPower_flg_fftinc
      link override fftlim: Value=KINP_PUIDLowPower_flg_fftlim
      link override invalid: Value=KINP_PUIDLowPower_flg_invalid
      link override ovrdflg: Value=KINP_PUIDLowPower_flg_ovrdflg
      link override ovrdval: Value=KINP_PUIDLowPower_flg_ovrdval
      link override setvalid: Value=KINP_PUIDLowPower_flg_setvalid
      link override srvcflg: Value=KINP_PUIDLowPower_flg_srvcflg
      link override srvcval: Value=KINP_PUIDLowPower_flg_srvcval
  Terminator_{1..12} (12 alike) : Terminator
  True_VHAL_DKCReVehData_enum : Constant  Value=TRUE  OutDataTypeStr=boolean
  True_VHAL_DKCRemotePW_enum : Constant  Value=TRUE  OutDataTypeStr=boolean
  True_VHAL_PCommandToBCM_enum : Constant  Value=TRUE  OutDataTypeStr=boolean
  True_VHAL_PCommandToPTG_enum : Constant  Value=TRUE  OutDataTypeStr=boolean
  True_VHAL_PDKeyAreaLockUnlock_enum : Constant  Value=TRUE  OutDataTypeStr=boolean
  True_VHAL_PDKeyAreaPS_enum : Constant  Value=TRUE  OutDataTypeStr=boolean
  True_VHAL_PDKeyAreaPTG_enum : Constant  Value=TRUE  OutDataTypeStr=boolean
  True_VHAL_PDKeyWelcome_enum : Constant  Value=TRUE  OutDataTypeStr=boolean
  True_VHAL_PDkeyShowIVI_enum : Constant  Value=TRUE  OutDataTypeStr=boolean
  True_VHAL_PKeyMiss_flg : Constant  Value=TRUE  OutDataTypeStr=boolean
  True_VHAL_PKeyMode_enum : Constant  Value=TRUE  OutDataTypeStr=boolean
  True_VHAL_PUIDLowPower_flg : Constant  Value=TRUE  OutDataTypeStr=boolean
  slr1_{1..12} (12 alike) : BusSelector  OutputSignals=VINP_CANMsgValidDKC1_flg
  slr_VHAL_DKCReVehData_enum : BusSelector  OutputSignals=VHAL_DKCReVehData_enum
  slr_VHAL_DKCRemotePW_enum : BusSelector  OutputSignals=VHAL_DKCRemotePW_enum
  slr_VHAL_PCommandToBCM_enum : BusSelector  OutputSignals=VHAL_PCommandToBCM_enum
  slr_VHAL_PCommandToPTG_enum : BusSelector  OutputSignals=VHAL_PCommandToPTG_enum
  slr_VHAL_PDKeyAreaLockUnlock_enum : BusSelector  OutputSignals=VHAL_PDKeyAreaLockUnlock_enum
  slr_VHAL_PDKeyAreaPS_enum : BusSelector  OutputSignals=VHAL_PDKeyAreaPS_enum
  slr_VHAL_PDKeyAreaPTG_enum : BusSelector  OutputSignals=VHAL_PDKeyAreaPTG_enum
  slr_VHAL_PDKeyWelcome_enum : BusSelector  OutputSignals=VHAL_PDKeyWelcome_enum
  slr_VHAL_PDkeyShowIVI_enum : BusSelector  OutputSignals=VHAL_PDkeyShowIVI_enum
  slr_VHAL_PKeyMiss_flg : BusSelector  OutputSignals=VHAL_PKeyMiss_flg
  slr_VHAL_PKeyMode_enum : BusSelector  OutputSignals=VHAL_PKeyMode_enum
  slr_VHAL_PUIDLowPower_flg : BusSelector  OutputSignals=VHAL_PUIDLowPower_flg
  VINP_DKCReVehData_enum : Outport
  VINP_DKCRemotePW_enum : Outport  Port=2
  VINP_PCommandToBCM_enum : Outport  Port=3
  VINP_PCommandToPTG_enum : Outport  Port=4
  VINP_PDKeyAreaLockUnlock_enum : Outport  Port=5
  VINP_PDKeyAreaPS_enum : Outport  Port=6
  VINP_PDKeyAreaPTG_enum : Outport  Port=7
  VINP_PDKeyWelcome_enum : Outport  Port=8
  VINP_PDkeyShowIVI_enum : Outport  Port=9
  VINP_PKeyMiss_flg : Outport  Port=10
  VINP_PKeyMode_enum : Outport  Port=11
  VINP_PUIDLowPower_flg : Outport  Port=12
  wires:
  BHAL_outputs/1 -> [BHAL_outputs]
  inp_CanValid_bus/1 -> [inp_CanValid_bus]
  [BHAL_outputs] -> slr_VHAL_DKCReVehData_enum/1
  slr_VHAL_DKCReVehData_enum/1 -> DKCReVehData/1  "<VHAL_DKCReVehData_enum>"
  True_VHAL_DKCReVehData_enum/1 -> DKCReVehData/2
  [inp_CanValid_bus] -> slr1_1/1
  slr1_1/1 -> DKCReVehData/3  "<VINP_CANMsgValidDKC1_flg>"
  DKCReVehData/1 -> VINP_DKCReVehData_enum/1  "VINP_DKCReVehData_enum"
  DKCReVehData/2 -> Terminator_1/1
  [BHAL_outputs] -> slr_VHAL_DKCRemotePW_enum/1
  slr_VHAL_DKCRemotePW_enum/1 -> DKCRemotePW/1  "<VHAL_DKCRemotePW_enum>"
  True_VHAL_DKCRemotePW_enum/1 -> DKCRemotePW/2
  [inp_CanValid_bus] -> slr1_2/1
  slr1_2/1 -> DKCRemotePW/3  "<VINP_CANMsgValidDKC1_flg>"
  DKCRemotePW/1 -> VINP_DKCRemotePW_enum/1  "VINP_DKCRemotePW_enum"
  DKCRemotePW/2 -> Terminator_2/1
  [BHAL_outputs] -> slr_VHAL_PCommandToBCM_enum/1
  slr_VHAL_PCommandToBCM_enum/1 -> PCommandToBCM/1  "<VHAL_PCommandToBCM_enum>"
  True_VHAL_PCommandToBCM_enum/1 -> PCommandToBCM/2
  [inp_CanValid_bus] -> slr1_3/1
  slr1_3/1 -> PCommandToBCM/3  "<VINP_CANMsgValidDKC1_flg>"
  PCommandToBCM/1 -> VINP_PCommandToBCM_enum/1  "VINP_PCommandToBCM_enum"
  PCommandToBCM/2 -> Terminator_3/1
  [BHAL_outputs] -> slr_VHAL_PCommandToPTG_enum/1
  slr_VHAL_PCommandToPTG_enum/1 -> PCommandToPTG/1  "<VHAL_PCommandToPTG_enum>"
  True_VHAL_PCommandToPTG_enum/1 -> PCommandToPTG/2
  [inp_CanValid_bus] -> slr1_4/1
  slr1_4/1 -> PCommandToPTG/3  "<VINP_CANMsgValidDKC1_flg>"
  PCommandToPTG/1 -> VINP_PCommandToPTG_enum/1  "VINP_PCommandToPTG_enum"
  PCommandToPTG/2 -> Terminator_4/1
  [BHAL_outputs] -> slr_VHAL_PDKeyAreaLockUnlock_enum/1
  slr_VHAL_PDKeyAreaLockUnlock_enum/1 -> PDKeyAreaLockUnlock/1  "<VHAL_PDKeyAreaLockUnlock_enum>"
  True_VHAL_PDKeyAreaLockUnlock_enum/1 -> PDKeyAreaLockUnlock/2
  [inp_CanValid_bus] -> slr1_5/1
  slr1_5/1 -> PDKeyAreaLockUnlock/3  "<VINP_CANMsgValidDKC1_flg>"
  PDKeyAreaLockUnlock/1 -> VINP_PDKeyAreaLockUnlock_enum/1  "VINP_PDKeyAreaLockUnlock_enum"
  PDKeyAreaLockUnlock/2 -> Terminator_5/1
  [BHAL_outputs] -> slr_VHAL_PDKeyAreaPS_enum/1
  slr_VHAL_PDKeyAreaPS_enum/1 -> PDKeyAreaPS/1  "<VHAL_PDKeyAreaPS_enum>"
  True_VHAL_PDKeyAreaPS_enum/1 -> PDKeyAreaPS/2
  [inp_CanValid_bus] -> slr1_6/1
  slr1_6/1 -> PDKeyAreaPS/3  "<VINP_CANMsgValidDKC1_flg>"
  PDKeyAreaPS/1 -> VINP_PDKeyAreaPS_enum/1  "VINP_PDKeyAreaPS_enum"
  PDKeyAreaPS/2 -> Terminator_6/1
  [BHAL_outputs] -> slr_VHAL_PDKeyAreaPTG_enum/1
  slr_VHAL_PDKeyAreaPTG_enum/1 -> PDKeyAreaPTG/1  "<VHAL_PDKeyAreaPTG_enum>"
  True_VHAL_PDKeyAreaPTG_enum/1 -> PDKeyAreaPTG/2
  [inp_CanValid_bus] -> slr1_7/1
  slr1_7/1 -> PDKeyAreaPTG/3  "<VINP_CANMsgValidDKC1_flg>"
  PDKeyAreaPTG/1 -> VINP_PDKeyAreaPTG_enum/1  "VINP_PDKeyAreaPTG_enum"
  PDKeyAreaPTG/2 -> Terminator_7/1
  [BHAL_outputs] -> slr_VHAL_PDKeyWelcome_enum/1
  slr_VHAL_PDKeyWelcome_enum/1 -> PDKeyWelcome/1  "<VHAL_PDKeyWelcome_enum>"
  True_VHAL_PDKeyWelcome_enum/1 -> PDKeyWelcome/2
  [inp_CanValid_bus] -> slr1_8/1
  slr1_8/1 -> PDKeyWelcome/3  "<VINP_CANMsgValidDKC1_flg>"
  PDKeyWelcome/1 -> VINP_PDKeyWelcome_enum/1  "VINP_PDKeyWelcome_enum"
  PDKeyWelcome/2 -> Terminator_8/1
  [BHAL_outputs] -> slr_VHAL_PDkeyShowIVI_enum/1
  slr_VHAL_PDkeyShowIVI_enum/1 -> PDkeyShowIVI/1  "<VHAL_PDkeyShowIVI_enum>"
  True_VHAL_PDkeyShowIVI_enum/1 -> PDkeyShowIVI/2
  [inp_CanValid_bus] -> slr1_9/1
  slr1_9/1 -> PDkeyShowIVI/3  "<VINP_CANMsgValidDKC1_flg>"
  PDkeyShowIVI/1 -> VINP_PDkeyShowIVI_enum/1  "VINP_PDkeyShowIVI_enum"
  PDkeyShowIVI/2 -> Terminator_9/1
  [BHAL_outputs] -> slr_VHAL_PKeyMiss_flg/1
  slr_VHAL_PKeyMiss_flg/1 -> PKeyMiss/1  "<VHAL_PKeyMiss_flg>"
  True_VHAL_PKeyMiss_flg/1 -> PKeyMiss/2
  [inp_CanValid_bus] -> slr1_10/1
  slr1_10/1 -> PKeyMiss/3  "<VINP_CANMsgValidDKC1_flg>"
  PKeyMiss/1 -> VINP_PKeyMiss_flg/1  "VINP_PKeyMiss_flg"
  PKeyMiss/2 -> Terminator_10/1
  [BHAL_outputs] -> slr_VHAL_PKeyMode_enum/1
  slr_VHAL_PKeyMode_enum/1 -> PKeyMode/1  "<VHAL_PKeyMode_enum>"
  True_VHAL_PKeyMode_enum/1 -> PKeyMode/2
  [inp_CanValid_bus] -> slr1_11/1
  slr1_11/1 -> PKeyMode/3  "<VINP_CANMsgValidDKC1_flg>"
  PKeyMode/1 -> VINP_PKeyMode_enum/1  "VINP_PKeyMode_enum"
  PKeyMode/2 -> Terminator_11/1
  [BHAL_outputs] -> slr_VHAL_PUIDLowPower_flg/1
  slr_VHAL_PUIDLowPower_flg/1 -> PUIDLowPower/1  "<VHAL_PUIDLowPower_flg>"
  True_VHAL_PUIDLowPower_flg/1 -> PUIDLowPower/2
  [inp_CanValid_bus] -> slr1_12/1
  slr1_12/1 -> PUIDLowPower/3  "<VINP_CANMsgValidDKC1_flg>"
  PUIDLowPower/1 -> VINP_PUIDLowPower_flg/1  "VINP_PUIDLowPower_flg"
  PUIDLowPower/2 -> Terminator_12/1

== system inp/INP/CAN4/SignalCheck/DKC2 ==
  BHAL_outputs : Inport
  inp_CanValid_bus : Inport  Port=2
  EncryptionDATA063 : FVT_lib/inp/can_signal_template  SystemSampleTime=-1  VariantActivationTime=update diagram  Latency=0  AutoFrameSizeCalculation=off
      link override defval: Value=KINP_EncryptionDATA063_enum_defval
      link override fftdec: Value=KINP_EncryptionDATA063_enum_fftdec
      link override fftinc: Value=KINP_EncryptionDATA063_enum_fftinc
      link override fftlim: Value=KINP_EncryptionDATA063_enum_fftlim
      link override invalid: Value=KINP_EncryptionDATA063_enum_invalid
      link override ovrdflg: Value=KINP_EncryptionDATA063_enum_ovrdflg
      link override ovrdval: Value=KINP_EncryptionDATA063_enum_ovrdval
      link override setvalid: Value=KINP_EncryptionDATA063_enum_setvalid
      link override srvcflg: Value=KINP_EncryptionDATA063_enum_srvcflg
      link override srvcval: Value=KINP_EncryptionDATA063_enum_srvcval
  EncryptionDATA64127 : FVT_lib/inp/can_signal_template  SystemSampleTime=-1  VariantActivationTime=update diagram  Latency=0  AutoFrameSizeCalculation=off
      link override defval: Value=KINP_EncryptionDATA64127_enum_defval
      link override fftdec: Value=KINP_EncryptionDATA64127_enum_fftdec
      link override fftinc: Value=KINP_EncryptionDATA64127_enum_fftinc
      link override fftlim: Value=KINP_EncryptionDATA64127_enum_fftlim
      link override invalid: Value=KINP_EncryptionDATA64127_enum_invalid
      link override ovrdflg: Value=KINP_EncryptionDATA64127_enum_ovrdflg
      link override ovrdval: Value=KINP_EncryptionDATA64127_enum_ovrdval
      link override setvalid: Value=KINP_EncryptionDATA64127_enum_setvalid
      link override srvcflg: Value=KINP_EncryptionDATA64127_enum_srvcflg
      link override srvcval: Value=KINP_EncryptionDATA64127_enum_srvcval
  RandomNumberX : FVT_lib/inp/can_signal_template  SystemSampleTime=-1  VariantActivationTime=update diagram  Latency=0  AutoFrameSizeCalculation=off
      link override defval: Value=KINP_RandomNumberX_enum_defval
      link override fftdec: Value=KINP_RandomNumberX_enum_fftdec
      link override fftinc: Value=KINP_RandomNumberX_enum_fftinc
      link override fftlim: Value=KINP_RandomNumberX_enum_fftlim
      link override invalid: Value=KINP_RandomNumberX_enum_invalid
      link override ovrdflg: Value=KINP_RandomNumberX_enum_ovrdflg
      link override ovrdval: Value=KINP_RandomNumberX_enum_ovrdval
      link override setvalid: Value=KINP_RandomNumberX_enum_setvalid
      link override srvcflg: Value=KINP_RandomNumberX_enum_srvcflg
      link override srvcval: Value=KINP_RandomNumberX_enum_srvcval
  Terminator_1 : Terminator
  Terminator_2 : Terminator
  Terminator_3 : Terminator
  True_VHAL_EncryptionDATA063_enum : Constant  Value=TRUE  OutDataTypeStr=boolean
  True_VHAL_EncryptionDATA64127_enum : Constant  Value=TRUE  OutDataTypeStr=boolean
  True_VHAL_RandomNumberX_enum : Constant  Value=TRUE  OutDataTypeStr=boolean
  slr1_1 : BusSelector  OutputSignals=VINP_CANMsgValidDKC2_flg
  slr1_2 : BusSelector  OutputSignals=VINP_CANMsgValidDKC2_flg
  slr1_3 : BusSelector  OutputSignals=VINP_CANMsgValidDKC2_flg
  slr_VHAL_EncryptionDATA063_enum : BusSelector  OutputSignals=VHAL_EncryptionDATA063_enum
  slr_VHAL_EncryptionDATA64127_enum : BusSelector  OutputSignals=VHAL_EncryptionDATA64127_enum
  slr_VHAL_RandomNumberX_enum : BusSelector  OutputSignals=VHAL_RandomNumberX_enum
  VINP_EncryptionDATA063_enum : Outport
  VINP_EncryptionDATA64127_enum : Outport  Port=2
  VINP_RandomNumberX_enum : Outport  Port=3
  wires:
  BHAL_outputs/1 -> [BHAL_outputs]
  inp_CanValid_bus/1 -> [inp_CanValid_bus]
  [BHAL_outputs] -> slr_VHAL_EncryptionDATA063_enum/1
  slr_VHAL_EncryptionDATA063_enum/1 -> EncryptionDATA063/1  "<VHAL_EncryptionDATA063_enum>"
  True_VHAL_EncryptionDATA063_enum/1 -> EncryptionDATA063/2
  [inp_CanValid_bus] -> slr1_1/1
  slr1_1/1 -> EncryptionDATA063/3  "<VINP_CANMsgValidDKC2_flg>"
  EncryptionDATA063/1 -> VINP_EncryptionDATA063_enum/1  "VINP_EncryptionDATA063_enum"
  EncryptionDATA063/2 -> Terminator_1/1
  [BHAL_outputs] -> slr_VHAL_EncryptionDATA64127_enum/1
  slr_VHAL_EncryptionDATA64127_enum/1 -> EncryptionDATA64127/1  "<VHAL_EncryptionDATA64127_enum>"
  True_VHAL_EncryptionDATA64127_enum/1 -> EncryptionDATA64127/2
  [inp_CanValid_bus] -> slr1_2/1
  slr1_2/1 -> EncryptionDATA64127/3  "<VINP_CANMsgValidDKC2_flg>"
  EncryptionDATA64127/1 -> VINP_EncryptionDATA64127_enum/1  "VINP_EncryptionDATA64127_enum"
  EncryptionDATA64127/2 -> Terminator_2/1
  [BHAL_outputs] -> slr_VHAL_RandomNumberX_enum/1
  slr_VHAL_RandomNumberX_enum/1 -> RandomNumberX/1  "<VHAL_RandomNumberX_enum>"
  True_VHAL_RandomNumberX_enum/1 -> RandomNumberX/2
  [inp_CanValid_bus] -> slr1_3/1
  slr1_3/1 -> RandomNumberX/3  "<VINP_CANMsgValidDKC2_flg>"
  RandomNumberX/1 -> VINP_RandomNumberX_enum/1  "VINP_RandomNumberX_enum"
  RandomNumberX/2 -> Terminator_3/1

== system inp/INP/CAN4/SignalCheck/GW_ZDR_PTG1 ==
  BHAL_outputs : Inport
  inp_CanValid_bus : Inport  Port=2
  PTGRDILSta : FVT_lib/inp/can_signal_template  SystemSampleTime=-1  VariantActivationTime=update diagram  Latency=0  AutoFrameSizeCalculation=off
      link override defval: Value=KINP_PTGRDILSta_enum_defval
      link override fftdec: Value=KINP_PTGRDILSta_enum_fftdec
      link override fftinc: Value=KINP_PTGRDILSta_enum_fftinc
      link override fftlim: Value=KINP_PTGRDILSta_enum_fftlim
      link override invalid: Value=KINP_PTGRDILSta_enum_invalid
      link override ovrdflg: Value=KINP_PTGRDILSta_enum_ovrdflg
      link override ovrdval: Value=KINP_PTGRDILSta_enum_ovrdval
      link override setvalid: Value=KINP_PTGRDILSta_enum_setvalid
      link override srvcflg: Value=KINP_PTGRDILSta_enum_srvcflg
      link override srvcval: Value=KINP_PTGRDILSta_enum_srvcval
  Terminator_1 : Terminator
  True_VHAL_PTGRDILSta_enum : Constant  Value=TRUE  OutDataTypeStr=boolean
  slr1_1 : BusSelector  OutputSignals=VINP_CANMsgValidGWZDRPTG1_flg
  slr_VHAL_PTGRDILSta_enum : BusSelector  OutputSignals=VHAL_PTGRDILSta_enum
  VINP_PTGRDILSta_enum : Outport
  wires:
  BHAL_outputs/1 -> [BHAL_outputs]
  inp_CanValid_bus/1 -> [inp_CanValid_bus]
  [BHAL_outputs] -> slr_VHAL_PTGRDILSta_enum/1
  slr_VHAL_PTGRDILSta_enum/1 -> PTGRDILSta/1  "<VHAL_PTGRDILSta_enum>"
  True_VHAL_PTGRDILSta_enum/1 -> PTGRDILSta/2
  [inp_CanValid_bus] -> slr1_1/1
  slr1_1/1 -> PTGRDILSta/3  "<VINP_CANMsgValidGWZDRPTG1_flg>"
  PTGRDILSta/1 -> VINP_PTGRDILSta_enum/1  "VINP_PTGRDILSta_enum"
  PTGRDILSta/2 -> Terminator_1/1
